simulink model "Octave"  (R2018a)
settings: Solver=VariableStepAuto  StartTime=0.0  StopTime=0.001  RelTol=1e-3
undefined symbols (not defined in the file or in its folder): fdesignblkfcn, G1, G2, G3, G4, G5, G6, G7, G8, gcbh, get, T
libraries: dspsrcs4 x1, dspxfrm3 x1, dspobslib x1
(part 1 of 2)
settings Model: Creator=Daniel  LastModifiedBy=Daniel

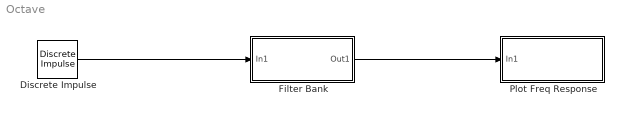
== system Octave ==
  Discrete Impulse : dspsrcs4/Discrete  Impulse  Delay=0  SampleTime=T  FrameSample=128  OutputFrames=off  dataType=double  isSigned=on  wordLen=16  udDataType=sfix(16)  fracBitsMode=Best precision  numFracBits=15  OutDataTypeStr=double  LastOutDataTypeStr=double
  "Filter Bank " : Subsystem
  Plot Freq Response : Subsystem
  wires:
  "Filter Bank "/1(Out1) -> Plot Freq Response/1(In1)
  Discrete Impulse/1 -> "Filter Bank "/1(In1)

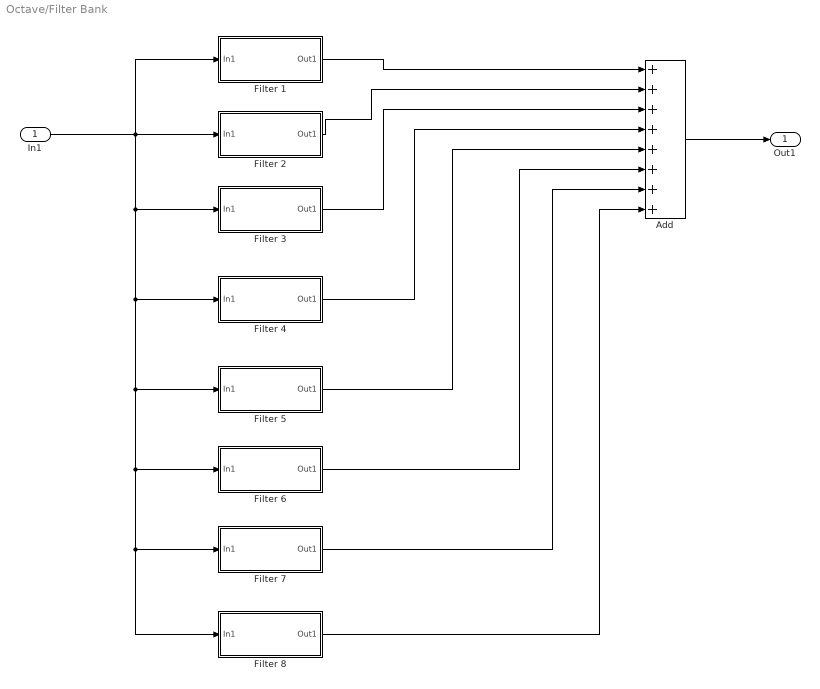
== system Octave/Filter Bank  ==
  In1 : Inport
  Add : Sum  Inputs=++++++++
  Filter 1 : Subsystem
  Filter 2 : Subsystem
  Filter 3 : Subsystem
  Filter 4 : Subsystem
  Filter 5 : Subsystem
  Filter 6 : Subsystem
  Filter 7 : Subsystem
  Filter 8 : Subsystem
  Out1 : Outport
  wires:
  In1/1 -> Filter 6/1(In1), Filter 8/1(In1), Filter 7/1(In1), Filter 5/1(In1), Filter 4/1(In1), Filter 3/1(In1), Filter 1/1(In1), Filter 2/1(In1)
  Add/1 -> Out1/1
  Filter 1/1(Out1) -> Add/1
  Filter 2/1(Out1) -> Add/2
  Filter 3/1(Out1) -> Add/3
  Filter 4/1(Out1) -> Add/4
  Filter 5/1(Out1) -> Add/5
  Filter 6/1(Out1) -> Add/6
  Filter 7/1(Out1) -> Add/7
  Filter 8/1(Out1) -> Add/8

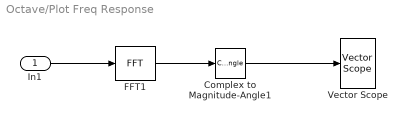
== system Octave/Plot Freq Response ==
  In1 : Inport
  Complex to Magnitude-Angle1 : ComplexToMagnitudeAngle  Output=Magnitude
  FFT1 : dspxfrm3/FFT  FFTImplementation=Auto  CompMethod=Table lookup  TableOpt=NEW  TableOptActive=Speed  BitRevOrder=off  Normalize=off  InheritFFTLength=on  FFTLength=64  WrapInput=on  roundingMode=Floor  overflowMode=off  firstCoeffDataTypeStr=Inherit: Same word length as input  firstCoeffLastDataTypeStr=Inherit: Same word length as input  outputMin=[]  outputMax=[]
  Vector Scope : dspobslib/Vector Scope  ScopeProperties=off  Domain=Frequency  HorizSpan=1  DisplayProperties=off  AxisGrid=on  Memory=off  FrameNumber=off  AxisLegend=off  AxisZoom=off  OpenScopeAtSimStart=on  OpenScopeImmediately=off  FigPos=get(0,'defaultfigureposition')  AxisProperties=on  XUnits=Hertz  XRange=[0...Fs/2]  InheritXIncr=on  XIncr=1  XLabel=Samples  XLimit=Auto  XMin=0  XMax=1  XStart=0  YUnits=dB  YLabel=|Magnitude (dB)|  LineProperties=off  XAxisParamsVer=6.9
      settings: SourceProductName=DSP System Toolbox  SourceProductBaseCode=DS  YMin=0.0723692553519949  YMax=69.3188381671759
  wires:
  In1/1 -> FFT1/1
  FFT1/1 -> Complex to Magnitude-Angle1/1
  Complex to Magnitude-Angle1/1 -> Vector Scope/1

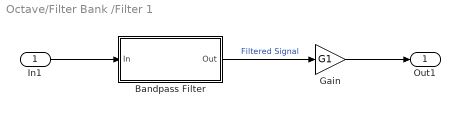
== system Octave/Filter Bank /Filter 1 ==
  In1 : Inport
  Bandpass Filter : Subsystem  DialogController=fdesignblkfcn  InitFcn=fdesignblkfcn(gcbh, {'InitFcn'});  mask(Bandpass Filter){}
      mask help: Design a bandpass filter
      settings: CopyFcn=fdesignblkfcn(gcbh, {'CopyFcn'});
      mask Help: helpview(mapfilelocation('dsp'), 'dspbandpassfilter');
      mask Display: disp('Bandpass');
  Gain : Gain  Gain=G1
  Out1 : Outport
  wires:
  Bandpass Filter/1(Out) -> Gain/1  "Filtered Signal"
  In1/1 -> Bandpass Filter/1(In)
  Gain/1 -> Out1/1

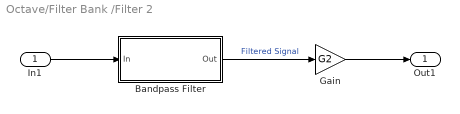
== system Octave/Filter Bank /Filter 2 ==
  In1 : Inport
  Bandpass Filter : Subsystem  DialogController=fdesignblkfcn  InitFcn=fdesignblkfcn(gcbh, {'InitFcn'});  mask(Bandpass Filter){}
      mask help: Design a bandpass filter
      settings: CopyFcn=fdesignblkfcn(gcbh, {'CopyFcn'});
      mask Help: helpview(mapfilelocation('dsp'), 'dspbandpassfilter');
      mask Display: disp('Bandpass');
  Gain : Gain  Gain=G2
  Out1 : Outport
  wires:
  Bandpass Filter/1(Out) -> Gain/1  "Filtered Signal"
  In1/1 -> Bandpass Filter/1(In)
  Gain/1 -> Out1/1

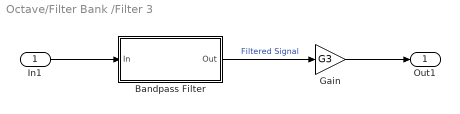
== system Octave/Filter Bank /Filter 3 ==
  In1 : Inport
  Bandpass Filter : Subsystem  DialogController=fdesignblkfcn  InitFcn=fdesignblkfcn(gcbh, {'InitFcn'});  mask(Bandpass Filter){}
      mask help: Design a bandpass filter
      settings: CopyFcn=fdesignblkfcn(gcbh, {'CopyFcn'});
      mask Help: helpview(mapfilelocation('dsp'), 'dspbandpassfilter');
      mask Display: disp('Bandpass');
  Gain : Gain  Gain=G3
  Out1 : Outport
  wires:
  Bandpass Filter/1(Out) -> Gain/1  "Filtered Signal"
  In1/1 -> Bandpass Filter/1(In)
  Gain/1 -> Out1/1

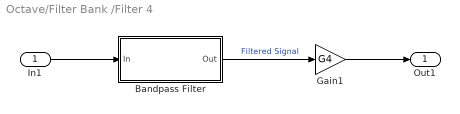
== system Octave/Filter Bank /Filter 4 ==
  In1 : Inport
  Bandpass Filter : Subsystem  DialogController=fdesignblkfcn  InitFcn=fdesignblkfcn(gcbh, {'InitFcn'});  mask(Bandpass Filter){}
      mask help: Design a bandpass filter
      settings: CopyFcn=fdesignblkfcn(gcbh, {'CopyFcn'});
      mask Help: helpview(mapfilelocation('dsp'), 'dspbandpassfilter');
      mask Display: disp('Bandpass');
  Gain1 : Gain  Gain=G4
  Out1 : Outport
  wires:
  Bandpass Filter/1(Out) -> Gain1/1  "Filtered Signal"
  In1/1 -> Bandpass Filter/1(In)
  Gain1/1 -> Out1/1

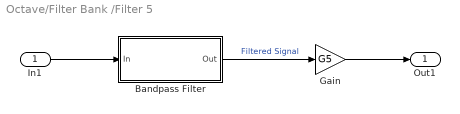
== system Octave/Filter Bank /Filter 5 ==
  In1 : Inport
  Bandpass Filter : Subsystem  DialogController=fdesignblkfcn  InitFcn=fdesignblkfcn(gcbh, {'InitFcn'});  mask(Bandpass Filter){}
      mask help: Design a bandpass filter
      settings: CopyFcn=fdesignblkfcn(gcbh, {'CopyFcn'});
      mask Help: helpview(mapfilelocation('dsp'), 'dspbandpassfilter');
      mask Display: disp('Bandpass');
  Gain : Gain  Gain=G5
  Out1 : Outport
  wires:
  Bandpass Filter/1(Out) -> Gain/1  "Filtered Signal"
  In1/1 -> Bandpass Filter/1(In)
  Gain/1 -> Out1/1

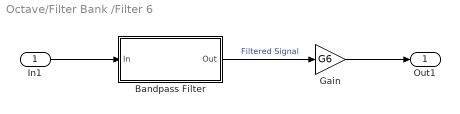
== system Octave/Filter Bank /Filter 6 ==
  In1 : Inport
  Bandpass Filter : Subsystem  DialogController=fdesignblkfcn  InitFcn=fdesignblkfcn(gcbh, {'InitFcn'});  mask(Bandpass Filter){}
      mask help: Design a bandpass filter
      settings: CopyFcn=fdesignblkfcn(gcbh, {'CopyFcn'});
      mask Help: helpview(mapfilelocation('dsp'), 'dspbandpassfilter');
      mask Display: disp('Bandpass');
  Gain : Gain  Gain=G6
  Out1 : Outport
  wires:
  Bandpass Filter/1(Out) -> Gain/1  "Filtered Signal"
  In1/1 -> Bandpass Filter/1(In)
  Gain/1 -> Out1/1

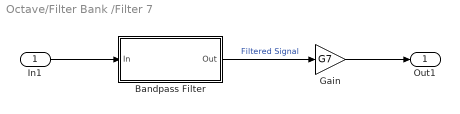
== system Octave/Filter Bank /Filter 7 ==
  In1 : Inport
  Bandpass Filter : Subsystem  DialogController=fdesignblkfcn  InitFcn=fdesignblkfcn(gcbh, {'InitFcn'});  mask(Bandpass Filter){}
      mask help: Design a bandpass filter
      settings: CopyFcn=fdesignblkfcn(gcbh, {'CopyFcn'});
      mask Help: helpview(mapfilelocation('dsp'), 'dspbandpassfilter');
      mask Display: disp('Bandpass');
  Gain : Gain  Gain=G7
  Out1 : Outport
  wires:
  Bandpass Filter/1(Out) -> Gain/1  "Filtered Signal"
  In1/1 -> Bandpass Filter/1(In)
  Gain/1 -> Out1/1

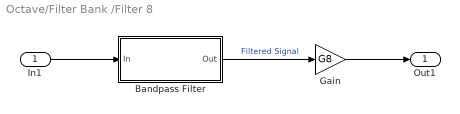
== system Octave/Filter Bank /Filter 8 ==
  In1 : Inport
  Bandpass Filter : Subsystem  DialogController=fdesignblkfcn  InitFcn=fdesignblkfcn(gcbh, {'InitFcn'});  mask(Bandpass Filter){}
      mask help: Design a bandpass filter
      settings: CopyFcn=fdesignblkfcn(gcbh, {'CopyFcn'});
      mask Help: helpview(mapfilelocation('dsp'), 'dspbandpassfilter');
      mask Display: disp('Bandpass');
  Gain : Gain  Gain=G8
  Out1 : Outport
  wires:
  Bandpass Filter/1(Out) -> Gain/1  "Filtered Signal"
  In1/1 -> Bandpass Filter/1(In)
  Gain/1 -> Out1/1

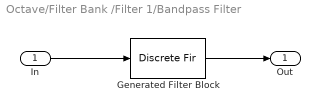
== system Octave/Filter Bank /Filter 1/Bandpass Filter ==
  In : Inport
  Generated Filter Block : DiscreteFir  Tag=BlockMethodSubSystem  Coefficients=[-0.306163146596753477 0.00372407254837170409 0.00366496521944481568 0.0036985371927436006 0.00364352519896121718 0.00368529200631995124 0.00363371291412095676 0.00368711368614621504 0.00363695818512055347 0.00370496574736567386 0.00365167005699301717 0.00374140966397434882 0.00367653903699310947 0.00380794349999374893 0.00370341665446805024 0.00400955205252634395 0.00341584839402697682 0.00361655794480864046 0.00398723703446579592 0.00394755699063087384 0.00407152445587033451 0.0040661178180966262 0.00414461614957689628 0.0041596319481752575 0.00422226706740808089 0.00425343188425031382 0.00430848667260652629 0.00435532951265332757 0.00440527028367487805 0.0044721726201434886 0.00451040270872937743 0.00462639515472151874 0.00463294931397623122 0.00458256912709448239 0.00479338636042297983 0.004838890610071922 0.00495385740613635273 0.00500249134506192128 0.00509813721858010105 0.00515178913610658817 0.00524190741804342331 0.00530145066012421839 0.00539024570678015014 0.00545581245032805695 0.00554579679635941458 0.00561886349052326262 0.00571069552307112982 0.00579064841549681297 0.00590811584580042126 0.00590543771033946729 0.00603848175711507729 0.0061307036884055699 0.00623947304517497026 0.00632190417658023973 0.00642082645328084789 0.00649875580932440799 0.00659362977855637578 0.00666984976654205752 0.00676293306031372499 0.00683804412716637611 0.00693134119210941924 0.00700672586682238308 0.00710400388393367388 0.00717522985441576555 0.0072889390730302428 0.00733359190744647949 0.00741266471686052864 0.0075057773930782834 0.00759404479951253375 0.00767577419461712429 0.00775696423222371756 0.00782972794463071553 0.00790508881474882852 0.00797171322369033541 0.00804258770280003032 0.00810396913956151765 0.00817160633617736165 0.00822970812562717757 0.00829858732997396098 0.00835461713240559511 0.00842588097120067214 0.00847603819761300059 0.0085145652567574226 0.00857433237564725337 0.00862949033227161655 0.00868339128277756389 0.00873245942492278937 0.00877741121409164604 0.00881909526381724485 0.00885656106234555818 0.00889168698423875581 0.008922337954022308 0.00895132831263767414 0.00897692958209000968 0.00900370762421065507 0.00903083038133917215 0.00905836486353139847 0.00907930385242833315 0.00908587835700336299 0.00909998021792990386 0.00911590117791671872 0.00913020832911953795 0.00914140303517457786 0.00914876738979975013 0.00915240212804729891 0.00915240212804729891 0.00914876738979975013 0.00914140303517457786 0.00913020832911953795 0.00911590117791671872 0.00909998021792990386 0.00908587835700336299 0.00907930385242833315 0.00905836486353139847 0.00903083038133917215 0.00900370762421065507 0.00897692958209000968 0.00895132831263767414 0.008922337954022308 0.00889168698423875581 0.00885656106234555818 0.00881909526381724485 0.00877741121409164604 0.00873245942492278937 0.00868339128277756389 0.00862949033227161655 0.00857433237564725337 0.0085145652567574226 0.00847603819761300059 0.00842588097120067214 0.00835461713240559511 0.00829858732997396098 0.00822970812562717757 0.00817160633617736165 0.00810396913956151765 0.00804258770280003032 0.00797171322369033541 0.00790508881474882852 0.00782972794463071553 0.00775696423222371756 0.00767577419461712429 0.00759404479951253375 0.0075057773930782834 0.00741266471686052864 0.00733359190744647949 0.0072889390730302428 0.00717522985441576555 0.00710400388393367388 0.00700672586682238308 0.00693134119210941924 0.00683804412716637611 0.00676293306031372499 0.00666984976654205752 0.00659362977855637578 0.00649875580932440799 0.00642082645328084789 0.00632190417658023973 0.00623947304517497026 0.0061307036884055699 0.00603848175711507729 0.00590543771033946729 0.00590811584580042126 0.00579064841549681297 0.00571069552307112982 0.00561886349052326262 0.00554579679635941458 0.00545581245032805695 0.00539024570678015014 0.00530145066012421839 0.00524190741804342331 0.00515178913610658817 0.00509813721858010105 0.00500249134506192128 0.00495385740613635273 ...(+821 chars)]  InputProcessing=Columns as channels (frame based)
  Out : Outport
  wires:
  In/1 -> Generated Filter Block/1
  Generated Filter Block/1 -> Out/1

== system Octave/Filter Bank /Filter 2/Bandpass Filter ==
  In : Inport
  Generated Filter Block : DiscreteFir  Tag=BlockMethodSubSystem  Coefficients=[0.126325295759325495 -0.0117624411795437533 -0.011270973078605806 -0.0106661147578010485 -0.010204067504695713 -0.00962678541484696115 -0.00919446712484628392 -0.00864358759994857118 -0.00824151745417281423 -0.00771533045939534756 -0.00734493995778551234 -0.00684065948323214768 -0.00650512686718529576 -0.00601631000542193761 -0.00572578488868016877 -0.0052238334422478605 -0.00503473166963042118 -0.00458937610346185632 -0.00410712608612090468 -0.00394342499452235429 -0.00367823972882377892 -0.00336592572408431212 -0.00306463087038175153 -0.00273485012579333109 -0.00247925921985930886 -0.00219398082132479799 -0.0019955589738708257 -0.00174883445865467446 -0.00158645964860656963 -0.00135818514905039489 -0.00121508839197470575 -0.000993252359553831177 -0.000872922695228539602 -0.000631573103288679549 -0.000571599800697875082 -0.000356150811276434442 -0.000225736215275690322 -8.92685379580149263e-05 -2.59224726173457043e-05 0.000105099570534422648 0.000169630555525435156 0.000292979901657025588 0.000331839388813121028 0.000424616641963138086 0.000434596715639085085 0.000506948997195305617 0.000504729193126413067 0.000569069772257430051 0.000563041769849614848 0.000618821044082618066 0.000597330039591198458 0.000664191828057159039 0.000597439857984050082 0.0006463753011436979 0.000602514540418874756 0.000622146986371308053 0.000548954450604627331 0.000556392404756800296 0.000485795655308624008 0.000492604183137013152 0.000414253194285979509 0.00040583605840621706 0.000313387895957667473 0.000292748189234220968 0.000194930685806893322 0.00016724772100243368 7.06624544546119449e-05 3.18473124721607714e-05 -7.23450349015553051e-05 -0.000101130322688214314 -0.000230968664549385805 -0.000265043299004424915 -0.000378993012366352078 -0.000414621225777817015 -0.000535742395975757901 -0.000574181490656078264 -0.000689033835469865519 -0.000721911499565658366 -0.000835593250605087823 -0.00087339646794279413 -0.000992593023948301623 -0.00103419793981304742 -0.00115235644487621247 -0.00119407093083673255 -0.00130253577870914627 -0.00135000786480760082 -0.0014557773900550075 -0.00149137053383543994 -0.00160761062197453675 -0.001642751564017636 -0.00174687577675597394 -0.00177490326335263959 -0.00187863231477547465 -0.00190623852342791666 -0.00200459881957201769 -0.0020246769158902278 -0.00211714468222776175 -0.00213392014684882225 -0.00222455579380986812 -0.00223620168364246918 -0.00232063168901783246 -0.00232526768913840498 -0.00239532521276344945 -0.00240145471175093328 -0.00246432206836222356 -0.0024598311856951216 -0.00252496304867719235 -0.0025187499088862586 -0.00257424817209844781 -0.00255843810410366634 -0.00260905548087708716 -0.00259035980382169018 -0.00263551013117094279 -0.00260916526804663707 -0.00264685955082119562 -0.00261492038897406798 -0.00264978001169141608 -0.00261188198592696152 -0.002643796625665773 -0.00260018911799772545 -0.00262196193009914258 -0.00258148330517957159 -0.00259892910271664057 -0.00255254028450879744 -0.00257019769546532051 -0.00252405667313859716 -0.00253578746620838902 -0.00248267246514707884 -0.002489956001528848 -0.00243609345543252531 -0.00244146449267984567 -0.00238499710707579249 -0.00238613737555962158 -0.00232752961674509429 -0.00232815194728211439 -0.00226623278186352528 -0.00226809598920024724 -0.00220257867935530482 -0.00219836960265654136 -0.00213645743292795176 -0.00213076437883699676 -0.0020664412882525629 -0.0020612935906385299 -0.00199990168202673901 -0.00199386479574251152 -0.0019308154855930959 -0.00192427790154151013 -0.00186486258156740026 -0.00186146397317982215 -0.00180550358491565754 -0.00180214560930430645 -0.00174867163595290864 -0.0017474352283111394 -0.00169451238063508813 -0.0016986676390594313 -0.00164600890898228269 -0.00164942698959644196 -0.00160251429863256245 -0.00160923324941686374 -0.00156429310496050689 -0.00157410781724512394 -0.00153461805042978683 -0.00154754611011639898 -0.00150977280137226666 -0.00152434618633265351 -0.00149100627151757537 -0.00151005348601859768 ...(+31572 chars)]  InputProcessing=Columns as channels (frame based)
  Out : Outport
  wires:
  In/1 -> Generated Filter Block/1
  Generated Filter Block/1 -> Out/1
